simulink model "Question2B2Homework3_AkankshaMurali"  (R2023b)
settings: Solver=FixedStepAuto  StartTime=0.0  StopTime=60  FixedStep=0.0001  MaxStep=1e-3  RelTol=1e-3  AbsTol=1e-3
settings Model: Creator=User  LastModifiedBy=akank
settings DebuggingCC: AlgebraicLoopMsg=none  UnconnectedInputMsg=warning  UnconnectedOutputMsg=warning  UnconnectedLineMsg=warning
settings ModelReferenceCC: EnableRefExpFcnMdlSchedulingChecks=on
settings RTWCC: DLArmComputeVersion=19.05

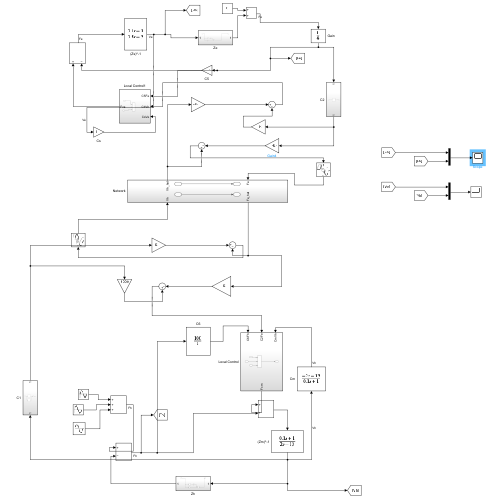
[thumbnail: Simulink's stored preview of the top-level diagram]
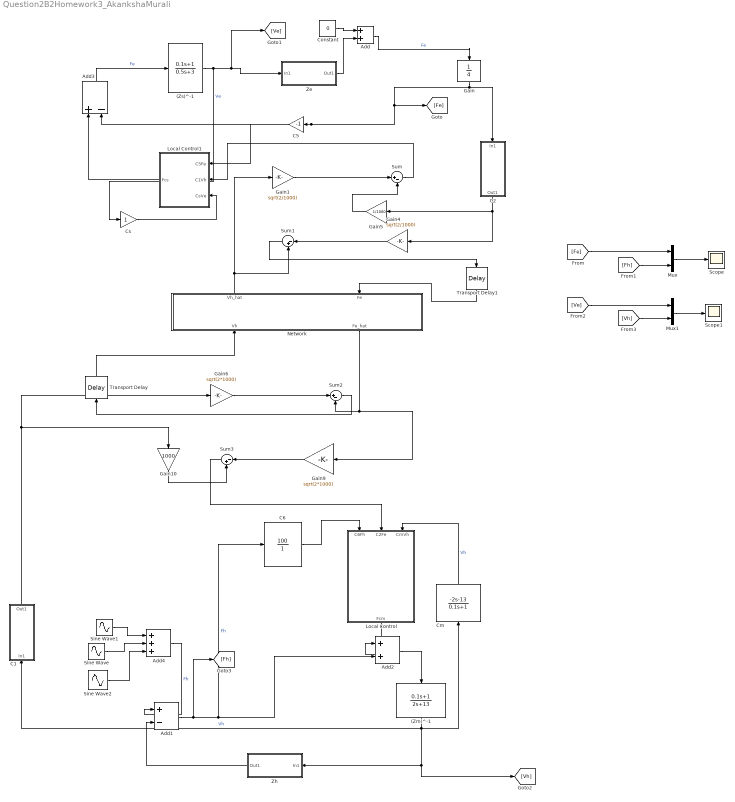
== system Question2B2Homework3_AkankshaMurali ==
  (Zm)^-1 : TransferFcn  Numerator=[0.1 1]  Denominator=[2 13]
  (Zs)^-1 : TransferFcn  Numerator=[0.1 1]  Denominator=[0.5 3]
  Add : Sum
  Add1 : Sum  Inputs=+-
  Add2 : Sum
  Add3 : Sum  Inputs=+-
  Add4 : Sum  Inputs=+++
  C1 : Subsystem
  C2 : Subsystem
  C5 : Gain  Gain=-1
  C6 : TransferFcn  Numerator=100  Denominator=1
  Cm : TransferFcn  Numerator=[-2 -13]  Denominator=[0.1 1]
  Constant : Constant  Value=0
  Cs : Gain
  Gain : TransferFcn  Numerator=1  Denominator=4
  Gain1 : Gain  Gain=sqrt(2/1000)
  Gain10 : Gain  Gain=1000
  Gain4 : Gain  Gain=sqrt(2/1000)
  Gain5 : Gain  Gain=1/1000
  Gain6 : Gain  Gain=sqrt(2*1000)
  Gain9 : Gain  Gain=sqrt(2*1000)
  Local Control : Subsystem
  Local Control1 : Subsystem
  Mux : Mux  Inputs=2
  Mux1 : Mux  Inputs=2
  Network : Subsystem
      settings: PortSchema="{\"entries\":[{\"content\":{\"sides\":[{\"content\":{\"connectorIds\":[\"Out2\",\"In1\"]},\"type\":\"ConnectorPlacement.EquallySpacedRectSide\",\"uuid\":\"46bbfd41-33ef-440b-a65b-3d407180442b\"},{\"content\":{\"connectorIds\":[\"In2\",\"Out1\"],\"side\":\"RIGHT\"},\"type\":\"ConnectorPlacement.EquallySpacedRectSide\",\"uuid\":\"e27f84dc-76da-44d4-b7d0-ad60a0198264\"},{\"content\":{\"connectorIds\":[],\"side\":\"TOP\"},\"type\":\"ConnectorPlacement.EquallySpacedRectSide\",\"uuid\":\"07067cb4-36f5-4d3d-827d-325a954000b1\"}]},\"type\":\"ConnectorPlacement.EquallySpacedConnector\",\"uuid\":\"c9856282-a0fe-4e0c-bbb9-ed49bb6b2e93\"}],\"packageUris\":[\"http://schema.mathworks.com/mf0/Connector/19700101\"],\"version\":\"1.0\"}"
  Scope : Scope
  Scope1 : Scope
  Sine Wave : Sin  Amplitude=20  Frequency=2  Phase=pi/2  SampleTime=0
  Sine Wave1 : Sin  Amplitude=20  SampleTime=0
  Sine Wave2 : Sin  Amplitude=20  Frequency=10  SampleTime=0
  Sum : Sum  Inputs=|+-
  Sum1 : Sum  Inputs=|-+
  Sum2 : Sum  Inputs=|+-
  Sum3 : Sum  Inputs=|-+
  Transport Delay : TransportDelay  DelayTime=0.1
  Transport Delay1 : TransportDelay  DelayTime=0.1
  Ze : Subsystem
  Zh : Subsystem
  wires:
  Ze/1(Out1) -> Add/2
  Add/1 -> Gain/1  "Fe"
  (Zm)^-1/1 -> Zh/1(In1), [Vh], C1/1(In1), Cm/1  "Vh"
  Cm/1 -> Local Control/3(CmVh)  "Vh"
  Zh/1(Out1) -> Add1/2
  Add1/1 -> C6/1, Add2/2, [Fh]  "Fh"
  C6/1 -> Local Control/1(C6Fh)
  Local Control/1(Fcm) -> Add2/1
  Add2/1 -> (Zm)^-1/1
  C5/1 -> Local Control1/1(C5Fe)
  Local Control1/1(Fcs) -> Add3/1
  Add3/1 -> (Zs)^-1/1  "Fe"
  (Zs)^-1/1 -> [Ve], Ze/1(In1), Cs/1  "Ve"
  Cs/1 -> Local Control1/3(CsVe)
  [Fe] -> Mux/1
  [Fh] -> Mux/2
  [Vh] -> Mux1/2
  [Ve] -> Mux1/1
  Sine Wave/1 -> Add4/2
  Sine Wave1/1 -> Add4/1
  Add4/1 -> Add1/1  "Fh"
  Mux1/1 -> Scope1/1
  Mux/1 -> Scope/1
  Constant/1 -> Add/1
  Sine Wave2/1 -> Add4/3
  Transport Delay1/1 -> Network/1(Fe)
  Transport Delay/1 -> Network/2(Vh)
  Sum2/1 -> Transport Delay/1
  Sum3/1 -> Local Control/2(C2Fe)
  Gain1/1 -> Sum/1
  Gain4/1 -> Sum1/1
  Network/2(Vh_hat) -> Sum1/2, Gain1/1
  Sum/1 -> Local Control1/2(C1Vh)
  Gain5/1 -> Sum/2
  Sum1/1 -> Transport Delay1/1
  Gain/1 -> C5/1, Add3/2, [Fe], C2/1(In1)
  Gain9/1 -> Sum3/1
  Gain6/1 -> Sum2/1
  Gain10/1 -> Sum3/2
  C2/1(Out1) -> Gain4/1, Gain5/1
  C1/1(Out1) -> Gain6/1, Gain10/1
  Network/1(Fe_hat) -> Gain9/1, Sum2/2

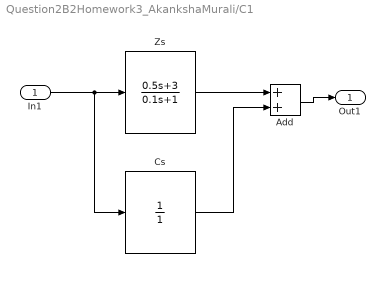
== system Question2B2Homework3_AkankshaMurali/C1 ==
  In1 : Inport
  Add : Sum
  Cs : TransferFcn  Numerator=1  Denominator=1
  Zs : TransferFcn  Numerator=[0.5 3]  Denominator=[0.1 1]
  Out1 : Outport
  wires:
  In1/1 -> Cs/1, Zs/1
  Cs/1 -> Add/2
  Zs/1 -> Add/1
  Add/1 -> Out1/1

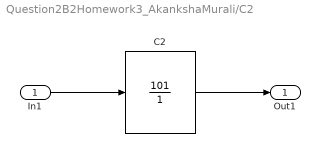
== system Question2B2Homework3_AkankshaMurali/C2 ==
  In1 : Inport
  C2 : TransferFcn  Numerator=101  Denominator=1
  Out1 : Outport
  wires:
  In1/1 -> C2/1
  C2/1 -> Out1/1

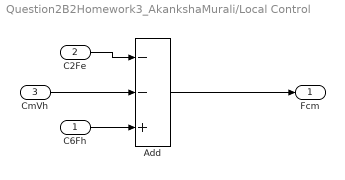
== system Question2B2Homework3_AkankshaMurali/Local Control ==
  C6Fh : Inport
  C2Fe : Inport  Port=2
  CmVh : Inport  Port=3
  Add : Sum  Inputs=--+
  Fcm : Outport
  wires:
  C2Fe/1 -> Add/1
  CmVh/1 -> Add/2
  C6Fh/1 -> Add/3
  Add/1 -> Fcm/1

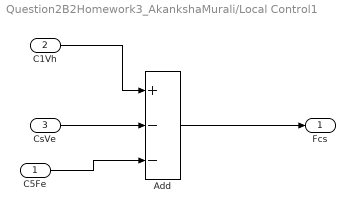
== system Question2B2Homework3_AkankshaMurali/Local Control1 ==
  C5Fe : Inport
  C1Vh : Inport  Port=2
  CsVe : Inport  Port=3
  Add : Sum  Inputs=+--
  Fcs : Outport
  wires:
  C5Fe/1 -> Add/3
  CsVe/1 -> Add/2
  C1Vh/1 -> Add/1
  Add/1 -> Fcs/1

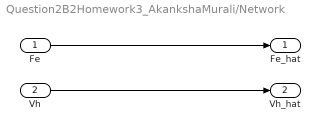
== system Question2B2Homework3_AkankshaMurali/Network ==
  Fe : Inport
  Vh : Inport  Port=2
  Fe_hat : Outport
  Vh_hat : Outport  Port=2
  wires:
  Fe/1 -> Fe_hat/1
  Vh/1 -> Vh_hat/1

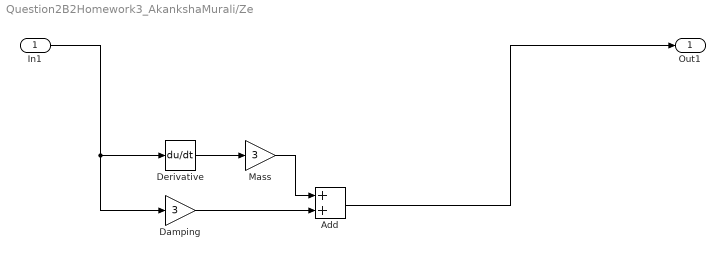
== system Question2B2Homework3_AkankshaMurali/Ze ==
  In1 : Inport
  Add : Sum
  Damping : Gain  Gain=3
  Derivative : Derivative
  Mass : Gain  Gain=3
  Out1 : Outport
  wires:
  Damping/1 -> Add/2
  Mass/1 -> Add/1
  In1/1 -> Damping/1, Derivative/1
  Derivative/1 -> Mass/1
  Add/1 -> Out1/1

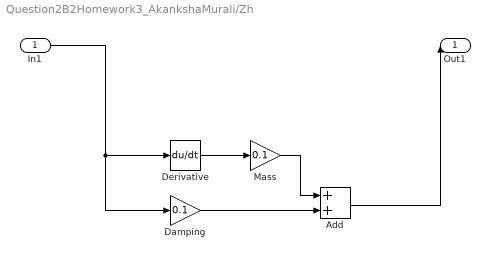
== system Question2B2Homework3_AkankshaMurali/Zh ==
  In1 : Inport
  Add : Sum
  Damping : Gain  Gain=0.1
  Derivative : Derivative
  Mass : Gain  Gain=0.1
  Out1 : Outport
  wires:
  In1/1 -> Damping/1, Derivative/1
  Derivative/1 -> Mass/1
  Damping/1 -> Add/2
  Mass/1 -> Add/1
  Add/1 -> Out1/1
